simulink model "Battery_model_2D_Battery2"  (R2026a)
settings: Solver=VariableStepAuto  StopTime=10000
InitFcn:
  | %% Universal Parameters
  | 
  | Cycle_num = 1000; % number of cycles
  | 
  | Temp_state = 35;
  | 
  | 
  | SoC_state = 0.5;
  | 
  | OCV = [ 3.0025,3.4635,3.521,3.5618,3.6058,3.6426,3.6725,3.7049,3.7486,3.79951,3.8418,3.8738 ,3.9044,3.9448,3.9813,4.0222 ,4.0498,4.0658,4.0919,4.1359,4.2];
  | 
  | 
  | % Cn = 540; % As
  | Ru = 3.19; % KW^-1
  | Rc = 1.94; % KW^-1
  | Cc = 62.7; % JK^-1
  | Cs = 4.5;  % JK^-1
  | 
  | Ea = 31500;  % J * mol^-1
  | eta = 152.5; % unitless
  | Ic = 9000;   % [1/s] normalized current rate
  | Rg = 8.314;  % J / K / mol
  | z = 0.57;    % Ah power law exponent
  | 
  | 
  | 
  | %% Breakpoints
  | Temp = [5, 15, 25, 35, 45];
  | SoC  = [0, 0.05, 0.10, 0.15, 0.20, 0.25, 0.30, 0.35, 0.40, 0.45, 0.50, 0.55, 0.60, 0.65, 0.70, 0.75, 0.80, 0.85, 0.90, 0.95, 1.00];
  | 
  | %% ── CHARGING Parameters ──────────────────────────────────────────────────────
  | %% CHARGING Parameters
  | 
  | % --- R0 (charge) ---
  | R0_5_ch  = [0.10039366, 0.10039366, 0.10039366, 0.08528700, 0.07769698, 0.08283688, 0.11006698 ...
  |              0.11427069, 0.11402639, 0.11444591, 0.11423324, 0.11397462, 0.11400530, 0.11412006 ...
  |              0.11437022, 0.11469884, 0.11501972, 0.11491341, 0.11445199, 0.11423824, 0.11366247];
  | R0_15_ch  = [0.13171649, 0.13171649, 0.13171649, 0.11189655, 0.10193844, 0.10868199, 0.14440788 ...
  |              0.14992315, 0.14960263, 0.15015303, 0.14987401, 0.14953470, 0.14957496, 0.14972552 ...
  |              0.15005372, 0.15048488, 0.15090588, 0.15076639, 0.15016101, 0.14988057, 0.14912516];
  | R0_25_ch  = [0.15680534, 0.15680534, 0.15680534, 0.13321018, 0.12135528, 0.12938332, 0.17191415 ...
  |              0.17847994, 0.17809836, 0.17875361, 0.17842144, 0.17801751, 0.17806543, 0.17824467 ...
  |              0.17863539, 0.17914866, 0.17964985, 0.17948380, 0.17876310, 0.17842925, 0.17752995];
  | R0_35_ch  = [0.18293956, 0.18293956, 0.18293956, 0.15541187, 0.14158117, 0.15094720, 0.20056650 ...
  |              0.20822660, 0.20778142, 0.20854588, 0.20815835, 0.20768709, 0.20774300, 0.20795212 ...
  |              0.20840795, 0.20900677, 0.20959150, 0.20939777, 0.20855695, 0.20816746, 0.20711828];
  | R0_45_ch  = [0.20580701, 0.20580701, 0.20580701, 0.17483836, 0.15927881, 0.16981560, 0.22563732 ...
  |              0.23425492, 0.23375410, 0.23461411, 0.23417814, 0.23364798, 0.23371087, 0.23394613 ...
  |              0.23445894, 0.23513262, 0.23579043, 0.23557249, 0.23462657, 0.23418839, 0.23300807];
  | R0_ch = [R0_5_ch; R0_15_ch; R0_25_ch; R0_35_ch; R0_45_ch];
  | 
  | % --- R1 (charge) ---
  | R1_5_ch  = [0.04985788, 0.04985788, 0.05071229, 0.04160410, 0.03661133, 0.03925367, 0.05381930 ...
  |              0.05642225, 0.05603500, 0.05496214, 0.05471562, 0.05430091, 0.05382478, 0.05367572 ...
  |              0.05355262, 0.05341750, 0.05337771, 0.05361159, 0.05382278, 0.05411150, 0.05453301];
  | R1_15_ch  = [0.07380278, 0.07380278, 0.07506754, 0.06158502, 0.05419440, 0.05810577, 0.07966673 ...
  |              0.08351978, 0.08294655, 0.08135843, 0.08099351, 0.08037963, 0.07967483, 0.07945418 ...
  |              0.07927196, 0.07907196, 0.07901306, 0.07935925, 0.07967188, 0.08009926, 0.08072321];
  | R1_25_ch  = [0.09348353, 0.09348353, 0.09508555, 0.07800769, 0.06864625, 0.07360064, 0.10091119 ...
  |              0.10579172, 0.10506563, 0.10305401, 0.10259178, 0.10181420, 0.10092146, 0.10064197 ...
  |              0.10041116, 0.10015782, 0.10008321, 0.10052172, 0.10091772, 0.10145906, 0.10224939];
  | R1_35_ch  = [0.14022529, 0.14022529, 0.14262832, 0.11701153, 0.10296937, 0.11040096, 0.15136678 ...
  |              0.15868759, 0.15759844, 0.15458101, 0.15388767, 0.15272130, 0.15138219, 0.15096295 ...
  |              0.15061673, 0.15023673, 0.15012481, 0.15078258, 0.15137658, 0.15218860, 0.15337409];
  | R1_45_ch  = [0.14957364, 0.14957364, 0.15213688, 0.12481230, 0.10983399, 0.11776102, 0.16145790 ...
  |              0.16926676, 0.16810500, 0.16488641, 0.16414685, 0.16290272, 0.16147433, 0.16102715 ...
  |              0.16065785, 0.16025251, 0.16013313, 0.16083476, 0.16146835, 0.16233450, 0.16359903];
  | R1_ch = [R1_5_ch; R1_15_ch; R1_25_ch; R1_35_ch; R1_45_ch];
  | 
  | % --- C1 (charge) ---
  | C1_5_ch  = [0.09227515, 0.09227515, 0.26008928, 0.33919625, 0.34687174, 0.30913179, 0.15915764 ...
  |              0.12842562, 0.12634235, 0.13107159, 0.12652827, 0.12226041, 0.12210630, 0.12333974 ...
  |              0.12544932, 0.12714870, 0.12951385, 0.13210182, 0.12944620, 0.12631334, 0.11822176];
  | C1_15_ch  = [0.08202235, 0.08202235, 0.23119047, 0.30150778, 0.30833043, 0.27478381, 0.14147345 ...
  |              0.11415611, 0.11230431, 0.11650808, 0.11246957, 0.10867592, 0.10853893, 0.10963532 ...
  |              0.11151051, 0.11302106, 0.11512343, 0.11742384, 0.11506329, 0.11227852, 0.10508601];
  | C1_25_ch  = [0.06561788, 0.06561788, 0.18495238, 0.24120622, 0.24666435, 0.21982705, 0.11317876 ...
  |              0.09132488, 0.08984345, 0.09320646, 0.08997566, 0.08694074, 0.08683115, 0.08770826 ...
  |              0.08920840, 0.09041685, 0.09209874, 0.09393907, 0.09205063, 0.08982282, 0.08406881];
  | C1_35_ch  = [0.06151676, 0.06151676, 0.17339285, 0.22613083, 0.23124783, 0.20608786, 0.10610509 ...
  |              0.08561708, 0.08422823, 0.08738106, 0.08435218, 0.08150694, 0.08140420, 0.08222649 ...
  |              0.08363288, 0.08476580, 0.08634257, 0.08806788, 0.08629747, 0.08420889, 0.07881451];
  | C1_45_ch  = [0.04921341, 0.04921341, 0.13871428, 0.18090467, 0.18499826, 0.16487029, 0.08488407 ...
  |              0.06849366, 0.06738259, 0.06990485, 0.06748174, 0.06520555, 0.06512336, 0.06578119 ...
  |              0.06690630, 0.06781264, 0.06907406, 0.07045431, 0.06903797, 0.06736711, 0.06305160];
  | C1_ch = [C1_5_ch; C1_15_ch; C1_25_ch; C1_35_ch; C1_45_ch];
  | 
  | % --- R2 (charge) ---
  | R2_5_ch  = [0.09089386, 0.09089386, 0.09135964, 0.07050606, 0.05920502, 0.06424266, 0.09305088 ...
  |              0.09755014, 0.09580263, 0.08885962, 0.08806550, 0.08655484, 0.08420777, 0.08313697 ...
  |              0.08166340, 0.07982229, 0.07868093, 0.07801613, 0.07782377, 0.07821878, 0.07934489];
  | R2_15_ch  = [0.12119181, 0.12119181, 0.12181285, 0.09400808, 0.07894002, 0.08565687, 0.12406784 ...
  |              0.13006685, 0.12773684, 0.11847950, 0.11742067, 0.11540645, 0.11227703, 0.11084930 ...
  |              0.10888454, 0.10642972, 0.10490791, 0.10402151, 0.10376502, 0.10429170, 0.10579318];
  | R2_25_ch  = [0.12832074, 0.12832074, 0.12897831, 0.09953796, 0.08358355, 0.09069551, 0.13136595 ...
  |              0.13771784, 0.13525077, 0.12544888, 0.12432777, 0.12219507, 0.11888156, 0.11736985 ...
  |              0.11528951, 0.11269029, 0.11107897, 0.11014042, 0.10986885, 0.11042651, 0.11201631];
  | R2_35_ch  = [0.16780404, 0.16780404, 0.16866394, 0.13016503, 0.10930157, 0.11860183, 0.17178624 ...
  |              0.18009256, 0.17686640, 0.16404853, 0.16258247, 0.15979355, 0.15546051, 0.15348364 ...
  |              0.15076320, 0.14736423, 0.14525711, 0.14402978, 0.14367465, 0.14440390, 0.14648287];
  | R2_45_ch  = [0.16780404, 0.16780404, 0.16866394, 0.13016503, 0.10930157, 0.11860183, 0.17178624 ...
  |              0.18009256, 0.17686640, 0.16404853, 0.16258247, 0.15979355, 0.15546051, 0.15348364 ...
  |              0.15076320, 0.14736423, 0.14525711, 0.14402978, 0.14367465, 0.14440390, 0.14648287];
  | R2_ch = [R2_5_ch; R2_15_ch; R2_25_ch; R2_35_ch; R2_45_ch];
  | 
  | % --- C2 (charge) ---
  | C2_5_ch  = [0.00983276, 0.00983276, 0.01035565, 0.01275571, 0.01321620, 0.01188380, 0.00709573 ...
  |              0.00612936, 0.00604375, 0.00608405, 0.00594967, 0.00578324, 0.00570466, 0.00570404 ...
  |              0.00576703, 0.00583752, 0.00589611, 0.00594399, 0.00590399, 0.00585441, 0.00573186];
  | C2_15_ch  = [0.00709364, 0.00709364, 0.00747086, 0.00920233, 0.00953455, 0.00857331, 0.00511907 ...
  |              0.00442190, 0.00436013, 0.00438920, 0.00429226, 0.00417219, 0.00411551, 0.00411505 ...
  |              0.00416050, 0.00421135, 0.00425362, 0.00428816, 0.00425931, 0.00422354, 0.00413513];
  | C2_25_ch  = [0.00584182, 0.00584182, 0.00615247, 0.00757839, 0.00785198, 0.00706038, 0.00421570 ...
  |              0.00364156, 0.00359070, 0.00361464, 0.00353480, 0.00343592, 0.00338924, 0.00338887 ...
  |              0.00342629, 0.00346817, 0.00350298, 0.00353143, 0.00350767, 0.00347821, 0.00340540];
  | C2_35_ch  = [0.00496555, 0.00496555, 0.00522960, 0.00644163, 0.00667418, 0.00600132, 0.00358335 ...
  |              0.00309533, 0.00305209, 0.00307244, 0.00300458, 0.00292054, 0.00288085, 0.00288054 ...
  |              0.00291235, 0.00294795, 0.00297754, 0.00300171, 0.00298152, 0.00295648, 0.00289459];
  | C2_45_ch  = [0.00381965, 0.00381965, 0.00402277, 0.00495510, 0.00513399, 0.00461640, 0.00275642 ...
  |              0.00238102, 0.00234776, 0.00236342, 0.00231122, 0.00224657, 0.00221604, 0.00221580 ...
  |              0.00224027, 0.00226765, 0.00229041, 0.00230901, 0.00229347, 0.00227421, 0.00222661];
  | C2_ch = [C2_5_ch; C2_15_ch; C2_25_ch; C2_35_ch; C2_45_ch];
  | 
  | %% DISCHARGING Parameters
  | 
  | % --- R0 (discharge) ---
  | R0_5_dis  = [0.10974667, 0.10974667, 0.10599493, 0.10491812, 0.10459081, 0.10424192, 0.10391050 ...
  |              0.10360923, 0.10340664, 0.10367370, 0.10378809, 0.10357423, 0.10367328, 0.10392792 ...
  |              0.10349265, 0.10276346, 0.10258047, 0.10278050, 0.10278050, 0.10278050, 0.10278050];
  | R0_15_dis  = [0.15445828, 0.15445828, 0.14917805, 0.14766253, 0.14720188, 0.14671085, 0.14624440 ...
  |              0.14582040, 0.14553527, 0.14591113, 0.14607213, 0.14577114, 0.14591054, 0.14626892 ...
  |              0.14565632, 0.14463005, 0.14437252, 0.14465404, 0.14465404, 0.14465404, 0.14465404];
  | R0_25_dis  = [0.18956243, 0.18956243, 0.18308216, 0.18122220, 0.18065686, 0.18005422, 0.17948176 ...
  |              0.17896140, 0.17861147, 0.17907275, 0.17927034, 0.17890094, 0.17907203, 0.17951186 ...
  |              0.17876003, 0.17750052, 0.17718445, 0.17752995, 0.17752995, 0.17752995, 0.17752995];
  | R0_35_dis  = [0.23168742, 0.23168742, 0.22376708, 0.22149380, 0.22080283, 0.22006627, 0.21936660 ...
  |              0.21873060, 0.21830291, 0.21886669, 0.21910819, 0.21865671, 0.21886581, 0.21940339 ...
  |              0.21848448, 0.21694508, 0.21655878, 0.21698106, 0.21698106, 0.21698106, 0.21698106];
  | R0_45_dis  = [0.26064835, 0.26064835, 0.25173797, 0.24918053, 0.24840318, 0.24757455, 0.24678743 ...
  |              0.24607192, 0.24559077, 0.24622503, 0.24649672, 0.24598880, 0.24622404, 0.24682881 ...
  |              0.24579504, 0.24406321, 0.24362862, 0.24410369, 0.24410369, 0.24410369, 0.24410369];
  | R0_dis = [R0_5_dis; R0_15_dis; R0_25_dis; R0_35_dis; R0_45_dis];
  | 
  | % --- R1 (discharge) ---
  | R1_5_dis  = [0.03959912, 0.03959912, 0.03910968, 0.03839708, 0.03719962, 0.03650035, 0.03573789 ...
  |              0.03550570, 0.03600486, 0.03635088, 0.03581701, 0.03524835, 0.03530531, 0.03537131 ...
  |              0.03514362, 0.03493837, 0.03506404, 0.03578729, 0.03578729, 0.03578729, 0.03578729];
  | R1_15_dis  = [0.07199840, 0.07199840, 0.07110850, 0.06981287, 0.06763567, 0.06636428, 0.06497798 ...
  |              0.06455582, 0.06546338, 0.06609252, 0.06512184, 0.06408791, 0.06419147, 0.06431147 ...
  |              0.06389749, 0.06352431, 0.06375280, 0.06506780, 0.06506780, 0.06506780, 0.06506780];
  | R1_25_dis  = [0.11314034, 0.11314034, 0.11174193, 0.10970594, 0.10628463, 0.10428672, 0.10210826 ...
  |              0.10144487, 0.10287103, 0.10385967, 0.10233432, 0.10070958, 0.10087230, 0.10106088 ...
  |              0.10041034, 0.09982391, 0.10018297, 0.10224939, 0.10224939, 0.10224939, 0.10224939];
  | R1_35_dis  = [0.15839648, 0.15839648, 0.15643871, 0.15358832, 0.14879848, 0.14600141, 0.14295156 ...
  |              0.14202281, 0.14401945, 0.14540354, 0.14326805, 0.14099341, 0.14122123, 0.14148523 ...
  |              0.14057447, 0.13975347, 0.14025616, 0.14314915, 0.14314915, 0.14314915, 0.14314915];
  | R1_45_dis  = [0.17999600, 0.17999600, 0.17777126, 0.17453218, 0.16908919, 0.16591069, 0.16244496 ...
  |              0.16138956, 0.16365846, 0.16523129, 0.16280460, 0.16021978, 0.16047867, 0.16077867 ...
  |              0.15974372, 0.15881076, 0.15938200, 0.16266949, 0.16266949, 0.16266949, 0.16266949];
  | R1_dis = [R1_5_dis; R1_15_dis; R1_25_dis; R1_35_dis; R1_45_dis];
  | 
  | % --- C1 (discharge) ---
  | C1_5_dis  = [0.25865012, 0.25865012, 0.25495567, 0.25151206, 0.24609499, 0.23971906, 0.22786518 ...
  |              0.22182597, 0.21445199, 0.21130782, 0.20864333, 0.20649971, 0.21349917, 0.22178481 ...
  |              0.21838854, 0.21060828, 0.20687447, 0.20176513, 0.20176513, 0.20176513, 0.20176513];
  | C1_15_dis  = [0.15519007, 0.15519007, 0.15297340, 0.15090724, 0.14765700, 0.14383143, 0.13671911 ...
  |              0.13309558, 0.12867119, 0.12678469, 0.12518600, 0.12389983, 0.12809950, 0.13307089 ...
  |              0.13103312, 0.12636497, 0.12412468, 0.12105908, 0.12105908, 0.12105908, 0.12105908];
  | C1_25_dis  = [0.10777088, 0.10777088, 0.10623153, 0.10479669, 0.10253958, 0.09988294, 0.09494383 ...
  |              0.09242749, 0.08935500, 0.08804493, 0.08693472, 0.08604155, 0.08895799, 0.09241034 ...
  |              0.09099522, 0.08775345, 0.08619769, 0.08406881, 0.08406881, 0.08406881, 0.08406881];
  | C1_35_dis  = [0.07917861, 0.07917861, 0.07804765, 0.07699349, 0.07533520, 0.07338338, 0.06975465 ...
  |              0.06790591, 0.06564857, 0.06468607, 0.06387041, 0.06321420, 0.06535689, 0.06789331 ...
  |              0.06685363, 0.06447192, 0.06332892, 0.06176484, 0.06176484, 0.06176484, 0.06176484];
  | C1_45_dis  = [0.06928128, 0.06928128, 0.06829170, 0.06736930, 0.06591830, 0.06421046, 0.06103532 ...
  |              0.05941767, 0.05744250, 0.05660031, 0.05588661, 0.05531242, 0.05718728, 0.05940665 ...
  |              0.05849693, 0.05641293, 0.05541280, 0.05404423, 0.05404423, 0.05404423, 0.05404423];
  | C1_dis = [C1_5_dis; C1_15_dis; C1_25_dis; C1_35_dis; C1_45_dis];
  | 
  | % --- R2 (discharge) ---
  | R2_5_dis  = [0.08531563, 0.08531563, 0.08615528, 0.08329853, 0.07783962, 0.07496095, 0.07307666 ...
  |              0.07262795, 0.07352909, 0.07429917, 0.07148713, 0.06823238, 0.06783005, 0.06755245 ...
  |              0.06633675, 0.06454005, 0.06447191, 0.06608962, 0.06608962, 0.06608962, 0.06608962];
  | R2_15_dis  = [0.11375417, 0.11375417, 0.11487370, 0.11106470, 0.10378615, 0.09994794, 0.09743555 ...
  |              0.09683727, 0.09803879, 0.09906556, 0.09531618, 0.09097651, 0.09044007, 0.09006993 ...
  |              0.08844900, 0.08605339, 0.08596255, 0.08811950, 0.08811950, 0.08811950, 0.08811950];
  | R2_25_dis  = [0.14460276, 0.14460276, 0.14602589, 0.14118395, 0.13193155, 0.12705246, 0.12385875 ...
  |              0.12309822, 0.12462558, 0.12593079, 0.12116463, 0.11564810, 0.11496619, 0.11449568 ...
  |              0.11243517, 0.10938991, 0.10927443, 0.11201631, 0.11201631, 0.11201631, 0.11201631];
  | R2_35_dis  = [0.17063126, 0.17063126, 0.17231055, 0.16659706, 0.15567923, 0.14992191, 0.14615332 ...
  |              0.14525590, 0.14705818, 0.14859834, 0.14297426, 0.13646476, 0.13566011, 0.13510490 ...
  |              0.13267350, 0.12908009, 0.12894383, 0.13217925, 0.13217925, 0.13217925, 0.13217925];
  | R2_45_dis  = [0.17063126, 0.17063126, 0.17231055, 0.16659706, 0.15567923, 0.14992191, 0.14615332 ...
  |              0.14525590, 0.14705818, 0.14859834, 0.14297426, 0.13646476, 0.13566011, 0.13510490 ...
  |              0.13267350, 0.12908009, 0.12894383, 0.13217925, 0.13217925, 0.13217925, 0.13217925];
  | R2_dis = [R2_5_dis; R2_15_dis; R2_25_dis; R2_35_dis; R2_45_dis];
  | 
  | % --- C2 (discharge) ---
  | C2_5_dis  = [0.00775836, 0.00775836, 0.00769594, 0.00737404, 0.00681760, 0.00637471, 0.00590764 ...
  |              0.00567197, 0.00566534, 0.00568421, 0.00559762, 0.00552599, 0.00558487, 0.00564889 ...
  |              0.00560911, 0.00554423, 0.00550375, 0.00544864, 0.00544864, 0.00544864, 0.00544864];
  | C2_15_dis  = [0.00646530, 0.00646530, 0.00641328, 0.00614503, 0.00568133, 0.00531226, 0.00492304 ...
  |              0.00472664, 0.00472112, 0.00473684, 0.00466468, 0.00460499, 0.00465406, 0.00470741 ...
  |              0.00467426, 0.00462019, 0.00458646, 0.00454054, 0.00454054, 0.00454054, 0.00454054];
  | C2_25_dis  = [0.00484897, 0.00484897, 0.00480996, 0.00460877, 0.00426100, 0.00398419, 0.00369228 ...
  |              0.00354498, 0.00354084, 0.00355263, 0.00349851, 0.00345374, 0.00349054, 0.00353056 ...
  |              0.00350569, 0.00346515, 0.00343985, 0.00340540, 0.00340540, 0.00340540, 0.00340540];
  | C2_35_dis  = [0.00258612, 0.00258612, 0.00256531, 0.00245801, 0.00227253, 0.00212490, 0.00196921 ...
  |              0.00189066, 0.00188845, 0.00189474, 0.00186587, 0.00184200, 0.00186162, 0.00188296 ...
  |              0.00186970, 0.00184808, 0.00183458, 0.00181621, 0.00181621, 0.00181621, 0.00181621];
  | C2_45_dis  = [0.00149199, 0.00149199, 0.00147999, 0.00141808, 0.00131108, 0.00122591, 0.00113609 ...
  |              0.00109076, 0.00108949, 0.00109312, 0.00107646, 0.00106269, 0.00107401, 0.00108633 ...
  |              0.00107868, 0.00106620, 0.00105841, 0.00104782, 0.00104782, 0.00104782, 0.00104782];
  | C2_dis = [C2_5_dis; C2_15_dis; C2_25_dis; C2_35_dis; C2_45_dis];
model workspace (MAT data in the model file):
  C_As = 150
  Cn = 150
  I_c = 1
  I_c_full_charged = 0.0333333333333
  Tc_state = 35.0044118318
  Ts_state = 35.0027406087
  V1_state = 0.00398713164124
  V2_state = 0.00927212980774
  V_cutoff = 3
  V_max = 4.2
  current_SoC = 0.996576803874
undefined symbols (not defined in the file): V1_ini
libraries: simulink x7
(part 1 of 2)
settings Model: Creator=vatan  LastModifiedBy=beaga
settings DebuggingCC: UnderspecifiedInitializationDetection=Classic
settings SimscapeCC: SimscapeNominalValues="[{\"value\":\"1\",\"unit\":\"A\"},{\"value\":\"1\",\"unit\":\"bar\"},{\"value\":\"1\",\"unit\":\"cm^2\"},{\"value\":\"1\",\"unit\":\"cm^3/s\"},{\"value\":\"1\",\"unit\":\"kJ/kg\"},{\"value\":\"1\",\"unit\":\"kW\"},{\"value\":\"1\",\"unit\":\"l\"},{\"value\":\"1\",\"unit\":\"N\"},{\"value\":\"1\",\"unit\":\"N*m\"},{\"value\":\"1\",\"unit\":\"V\"}]"  SimscapeLogType=none  SimscapeLogDataHistory=5000.0

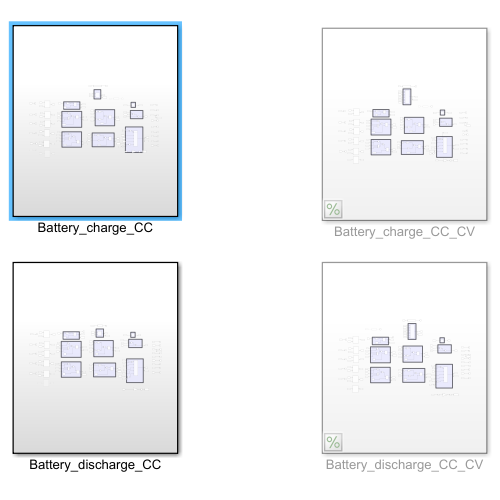
[thumbnail: Simulink's stored preview of the top-level diagram]
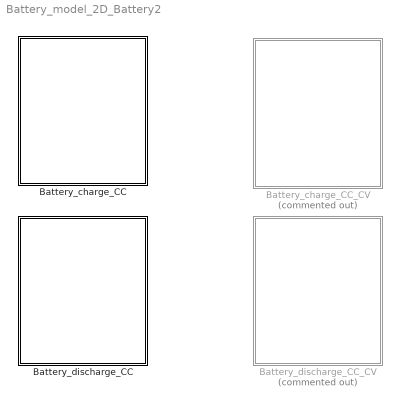
== system Battery_model_2D_Battery2 ==
  Battery_charge_CC : Subsystem
  Battery_charge_CC_CV : Subsystem  Commented=on
  Battery_discharge_CC : Subsystem
  Battery_discharge_CC_CV : Subsystem  Commented=on

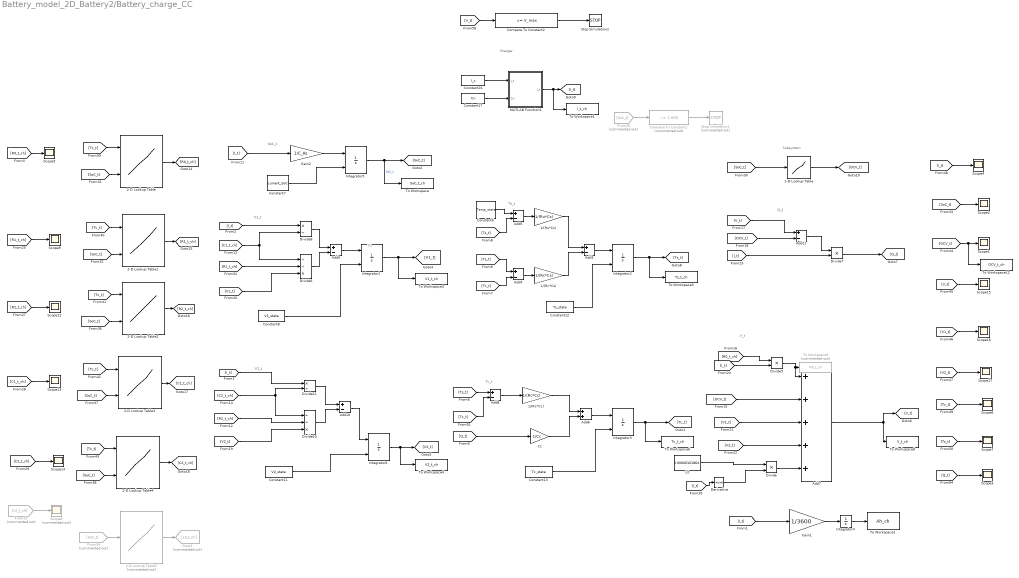
== system Battery_model_2D_Battery2/Battery_charge_CC ==
  note: Subsystem
  note: Tc_t
  note: Ts_t
  note: V_t
  note: V2_t
  note: V1_t
  note: SoC_t
  note: V1
  note: Q_t
  note: Charger
  1-D Lookup Table : Lookup_n-D  NumberOfTableDimensions=1  BreakpointsForDimension1=SoC  BreakpointsForDimension2=Temp  Table=OCV  InternalRulePriority=Speed  RndMeth=Simplest
  1/(Rc*Cc) : Gain  Gain=1/(Rc*Cc)
  1/(Rc*Cs) : Gain  Gain=1/(Rc*Cs)
  1/(Ru*Cs) : Gain  Gain=1/(Ru*Cs)
  2-D Lookup Table : Lookup_n-D  BreakpointsForDimension1=Temp  BreakpointsForDimension2=SoC  Table=R0_ch  InternalRulePriority=Speed  RndMeth=Simplest
      settings: InputPortMap=u0,u1
  2-D Lookup Table1 : Lookup_n-D  BreakpointsForDimension1=Temp  BreakpointsForDimension2=SoC  Table=R1_ch  InternalRulePriority=Speed  RndMeth=Simplest
      settings: InputPortMap=u0,u1
  2-D Lookup Table2 : Lookup_n-D  BreakpointsForDimension1=Temp  BreakpointsForDimension2=SoC  Table=R2_ch  InternalRulePriority=Speed  RndMeth=Simplest
      settings: InputPortMap=u0,u1
  2-D Lookup Table3 : Lookup_n-D  BreakpointsForDimension1=Temp  BreakpointsForDimension2=SoC  Table=C1_ch  InternalRulePriority=Speed  RndMeth=Simplest
      settings: InputPortMap=u0,u1
  2-D Lookup Table4 : Lookup_n-D  BreakpointsForDimension1=Temp  BreakpointsForDimension2=SoC  Table=C2_ch  InternalRulePriority=Speed  RndMeth=Simplest
      settings: InputPortMap=u0,u1
  2-D Lookup Table5 : Lookup_n-D  Commented=on  NumberOfTableDimensions=1  BreakpointsForDimension1=Temp  BreakpointsForDimension2=SoC  Table=C2_ch  InternalRulePriority=Speed  RndMeth=Simplest
  Add{3..5,8..11} (7 alike) : Sum  Inputs=+-
  Add6 : Sum
  Add7 : Sum  Inputs=+++++
  Cc : Gain  Gain=1/Cc
  Compare To Constant1 : simulink/Logic and Bit Operations/Compare To Constant  Commented=on  relop=~=  const=1.000  OutDataTypeStr=boolean
  Compare To Constant2 : simulink/Logic and Bit Operations/Compare To Constant  relop=>=  const=V_max  OutDataTypeStr=boolean
  Constant11 : Constant  Value=V2_state
  Constant12 : Constant  Value=Ts_state
  Constant13 : Constant  Value=Tc_state
  Constant16 : Constant  Value=I_c
  Constant17 : Constant  Value=Cn
  Constant6 : Constant  Value=Temp_state
  Constant7 : Constant  Value=current_SoC
  Constant8 : Constant  Value=V1_state
  Derivative : Derivative
  Divide : Product  Inputs=**
  Divide10 : Product  Inputs=//*
  Divide11 : Product  Inputs=*/
  Divide5 : Product  Inputs=**
  Divide6 : Product  Inputs=//*
  Divide7 : Product  Inputs=**
  Divide8 : Product  Inputs=*/
  From26 : From  Commented=on  GotoTag=SoC_t
  From34 : From  Commented=on  GotoTag=SoC_t
  From53 : From  Commented=on  GotoTag=L0_t_ch
  Gain1 : Gain  Gain=1/3600
  Gain2 : Gain  Gain=1/C_As
  Goto3 : Goto  Commented=on  GotoTag=L0_t_ch
  Integrator{1..3,6} (4 alike) : Integrator  InitialConditionSource=external
  Integrator4 : Integrator
  Integrator5 : Integrator  InitialConditionSource=external  InitialCondition=V1_ini
  L0 : Constant  Value=0.00000101864
  MATLAB Function4 : MATLAB Function  TreatAsAtomicUnit=on
  Scope{1..7,9,12..17} (14 alike) : Scope
      Scope1 settings: ActiveDisplayYMinimum=2.2604  ActiveDisplayYMaximum=3.6664  DataLoggingVariableName=ScopeData7
      Scope12 settings: ActiveDisplayYMinimum=0.00751  ActiveDisplayYMaximum=0.04204  DataLoggingVariableName=ScopeData3
      Scope13 settings: ActiveDisplayYMinimum=1446.0874  ActiveDisplayYMaximum=2982.5444  DataLoggingVariableName=ScopeData4
      Scope14 settings: ActiveDisplayYMinimum=14445.3812  ActiveDisplayYMaximum=112360.8817  DataLoggingVariableName=ScopeData5
      Scope15 settings: ActiveDisplayYMinimum=2.15  ActiveDisplayYMaximum=4.15  DataLoggingVariableName=ScopeData8
      Scope16 settings: ActiveDisplayYMinimum=-0.00306  ActiveDisplayYMaximum=0.0275  DataLoggingVariableName=ScopeData9
      Scope17 settings: ActiveDisplayYMinimum=-0.00274  ActiveDisplayYMaximum=0.02463  DataLoggingVariableName=ScopeData10
      Scope2 settings: ActiveDisplayYMinimum=0.0058466  ActiveDisplayYMaximum=0.025847  DataLoggingVariableName=ScopeData6
      Scope3 settings: ActiveDisplayYMinimum=-7.8351  ActiveDisplayYMaximum=6.6118  DataLoggingVariableName=ScopeData14
      Scope4 settings: ActiveDisplayYMinimum=0.049838  ActiveDisplayYMaximum=0.24984  DataLoggingVariableName=ScopeData11
      Scope5 settings: ActiveDisplayYMinimum=0.00753  ActiveDisplayYMaximum=0.01894
      Scope6 settings: ActiveDisplayYMinimum=24.9953  ActiveDisplayYMaximum=44.9953  DataLoggingVariableName=ScopeData12
      Scope7 settings: ActiveDisplayYMinimum=-5.0616  ActiveDisplayYMaximum=45.5546  DataLoggingVariableName=ScopeData13
      Scope9 settings: ActiveDisplayYMinimum=0.00821  ActiveDisplayYMaximum=0.03092  DataLoggingVariableName=ScopeData2
  Scope8 : Scope  Commented=on
      settings: ActiveDisplayYMinimum=14445.3812  ActiveDisplayYMaximum=112360.8817  DataLoggingVariableName=ScopeData24
  Stop Simulation1 : Stop  Commented=on
  Stop Simulation2 : Stop
  To Workspace : ToWorkspace  VariableName=SoC_t_ch  SampleTime=-1
      settings: Save2DSignal=2-D array (concatenate along first dimension)
  To Workspace1 : ToWorkspace  VariableName=I_t_ch  SaveFormat=Timeseries  SampleTime=-1
      settings: Save2DSignal=2-D array (concatenate along first dimension)
  To Workspace12 : ToWorkspace  VariableName=OCV_t_ch  SampleTime=-1
      settings: Save2DSignal=2-D array (concatenate along first dimension)
  To Workspace2 : ToWorkspace  VariableName=Ah_ch  SampleTime=-1
      settings: Save2DSignal=2-D array (concatenate along first dimension)
  To Workspace3 : ToWorkspace  VariableName=V1_t_ch  SampleTime=-1
      settings: Save2DSignal=2-D array (concatenate along first dimension)
  To Workspace4 : ToWorkspace  VariableName=V2_t_ch  SampleTime=-1
      settings: Save2DSignal=2-D array (concatenate along first dimension)
  To Workspace5 : ToWorkspace  VariableName=Ts_t_ch  SampleTime=-1
      settings: Save2DSignal=2-D array (concatenate along first dimension)
  To Workspace6 : ToWorkspace  VariableName=Tc_t_ch  SampleTime=-1
      settings: Save2DSignal=2-D array (concatenate along first dimension)
  To Workspace8 : ToWorkspace  VariableName=V_t_ch  SaveFormat=Timeseries  SampleTime=-1
      settings: Save2DSignal=2-D array (concatenate along first dimension)
  To Workspace9 : ToWorkspace  Commented=on  VariableName=R0_I_ch  SampleTime=-1
      settings: Save2DSignal=2-D array (concatenate along first dimension)
  wires:
  Divide10/1 -> Add10/2
  Add5/1 -> 1/(Ru*Cs)/1
  Add11/1 -> Divide7/1
  [Tc_t] -> Add4/2
  1/(Rc*Cc)/1 -> Add6/1
  [V2_t] -> Add7/4
  Divide5/1 -> Add7/1, To Workspace9/1
  Add4/1 -> 1/(Rc*Cs)/1
  Divide6/1 -> Add9/2
  [I_t] -> Divide11/1
  [Tc_t] -> 2-D Lookup Table2/1
  Cc/1 -> Add6/2
  [Tc_t] -> 2-D Lookup Table/1
  Divide7/1 -> [Q_t]
  1-D Lookup Table/1 -> [OCV_t]
  [SoC_t] -> 2-D Lookup Table1/2
  2-D Lookup Table3/1 -> [C1_t_ch]
  [V2_t] -> Scope17/1
  Add9/1 -> Integrator1/1
  2-D Lookup Table/1 -> [R0_t_ch]
  [Ts_t] -> Scope7/1
  [I_t] -> Scope4/1
  [V2_t] -> Divide10/3
  [R1_t_ch] -> Scope9/1
  Add10/1 -> Integrator6/1
  2-D Lookup Table4/1 -> [C2_t_ch]
  [SoC_t] -> 1-D Lookup Table/1
  [R0_t_ch] -> Scope5/1
  [SoC_t] -> 2-D Lookup Table/2
  [R0_t_ch] -> Divide5/1
  [I_t] -> Divide7/2
  [V1_t] -> Scope16/1
  [C2_t_ch] -> Divide10/1, Divide11/2
  Add3/1 -> Integrator2/1
  [V_t] -> Add11/1
  [Q_t] -> Scope3/1
  [I_t] -> Divide5/2
  [SoC_t] -> 2-D Lookup Table3/2
  1/(Rc*Cs)/1 -> Add3/2
  [OCV_t] -> To Workspace12/1, Scope1/1
  [C1_t_ch] -> Scope13/1
  [Tc_t] -> Scope6/1
  Divide8/1 -> Add9/1
  [OCV_t] -> Add11/2
  [V1_t] -> Divide6/3
  [Ts_t] -> Add4/1
  [Tc_t] -> 2-D Lookup Table1/1
  [C1_t_ch] -> Divide8/2, Divide6/1
  [Tc_t] -> 2-D Lookup Table3/1
  Gain2/1 -> Integrator5/1
  Add8/1 -> 1/(Rc*Cc)/1
  [R1_t_ch] -> Divide6/2
  [R2_t_ch] -> Scope12/1
  [Q_t] -> Cc/1
  Add6/1 -> Integrator3/1
  [R2_t_ch] -> Divide10/2
  [Ts_t] -> Add8/1
  2-D Lookup Table2/1 -> [R2_t_ch]
  Divide11/1 -> Add10/1
  [C2_t_ch] -> Scope14/1
  Add7/1 -> To Workspace8/1, [V_t]
  [SoC_t] -> 2-D Lookup Table2/2
  Integrator3/1 -> To Workspace6/1, [Tc_t]
  [Ts_t] -> Add5/2
  [Tc_t] -> Add8/2
  [I_t] -> Divide8/1
  Integrator6/1 -> To Workspace4/1, [V2_t]
  Integrator5/1 -> To Workspace/1, [SoC_t]  "SoC_t"
  Integrator1/1 -> To Workspace3/1, [V1_t]
  [SoC_t] -> Scope2/1
  Constant6/1 -> Add5/1
  2-D Lookup Table1/1 -> [R1_t_ch]
  [V_t] -> Scope15/1
  [SoC_t] -> 2-D Lookup Table4/2
  1/(Ru*Cs)/1 -> Add3/1
  [I_t] -> Gain2/1
  [Tc_t] -> 2-D Lookup Table4/1
  [OCV_t] -> Add7/2
  [V1_t] -> Add7/3
  [I_t] -> Gain1/1
  Integrator4/1 -> To Workspace2/1
  Gain1/1 -> Integrator4/1
  Integrator2/1 -> To Workspace5/1, [Ts_t]
  From26/1 -> Compare To Constant1/1
  Compare To Constant1/1 -> Stop Simulation1/1
  Constant12/1 -> Integrator2/2
  Constant8/1 -> Integrator1/2
  Constant11/1 -> Integrator6/2
  Constant13/1 -> Integrator3/2
  Constant16/1 -> MATLAB Function4/1(I_c)
  Constant17/1 -> MATLAB Function4/2(Cn)
  [V_t] -> Compare To Constant2/1
  Compare To Constant2/1 -> Stop Simulation2/1
  MATLAB Function4/1(I_t) -> To Workspace1/1, [I_t]
  Constant7/1 -> Integrator5/2
  From34/1 -> 2-D Lookup Table5/1
  2-D Lookup Table5/1 -> Goto3/1
  From53/1 -> Scope8/1
  [I_t] -> Derivative/1
  L0/1 -> Divide/1
  Derivative/1 -> Divide/2
  Divide/1 -> Add7/5

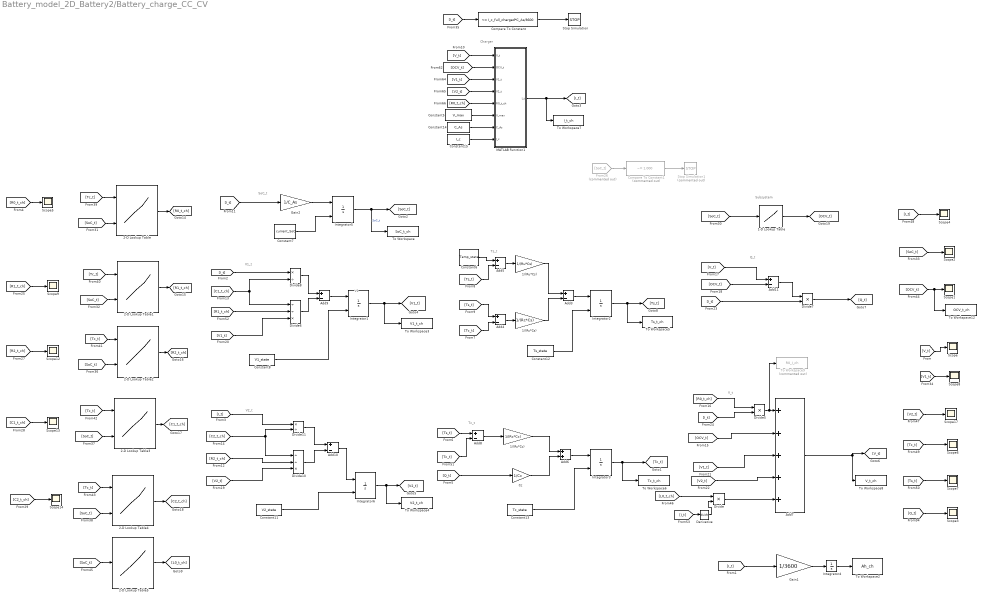
== system Battery_model_2D_Battery2/Battery_charge_CC_CV ==
  note: Subsystem
  note: Tc_t
  note: Ts_t
  note: V_t
  note: V2_t
  note: V1_t
  note: SoC_t
  note: V1
  note: Q_t
  note: Charger
  1-D Lookup Table : Lookup_n-D  NumberOfTableDimensions=1  BreakpointsForDimension1=SoC  BreakpointsForDimension2=Temp  Table=OCV  InternalRulePriority=Speed  RndMeth=Simplest
  1/(Rc*Cc) : Gain  Gain=1/(Rc*Cc)
  1/(Rc*Cs) : Gain  Gain=1/(Rc*Cs)
  1/(Ru*Cs) : Gain  Gain=1/(Ru*Cs)
  2-D Lookup Table : Lookup_n-D  BreakpointsForDimension1=Temp  BreakpointsForDimension2=SoC  Table=R0_ch  InternalRulePriority=Speed  RndMeth=Simplest
      settings: InputPortMap=u0,u1
  2-D Lookup Table1 : Lookup_n-D  BreakpointsForDimension1=Temp  BreakpointsForDimension2=SoC  Table=R1_ch  InternalRulePriority=Speed  RndMeth=Simplest
      settings: InputPortMap=u0,u1
  2-D Lookup Table2 : Lookup_n-D  BreakpointsForDimension1=Temp  BreakpointsForDimension2=SoC  Table=R2_ch  InternalRulePriority=Speed  RndMeth=Simplest
      settings: InputPortMap=u0,u1
  2-D Lookup Table3 : Lookup_n-D  BreakpointsForDimension1=Temp  BreakpointsForDimension2=SoC  Table=C1_ch  InternalRulePriority=Speed  RndMeth=Simplest
      settings: InputPortMap=u0,u1
  2-D Lookup Table4 : Lookup_n-D  BreakpointsForDimension1=Temp  BreakpointsForDimension2=SoC  Table=C2_ch  InternalRulePriority=Speed  RndMeth=Simplest
      settings: InputPortMap=u0,u1
  2-D Lookup Table5 : Lookup_n-D  NumberOfTableDimensions=1  BreakpointsForDimension1=Temp  BreakpointsForDimension2=SoC  Table=C2_ch  InternalRulePriority=Speed  RndMeth=Simplest
  Add{3..5,8..11} (7 alike) : Sum  Inputs=+-
  Add6 : Sum
  Add7 : Sum  Inputs=+++++
  Cc : Gain  Gain=1/Cc
  Compare To Constant : simulink/Logic and Bit Operations/Compare To Constant  relop=<=  const=I_c_full_charged*C_As/3600  OutDataTypeStr=boolean
  Compare To Constant1 : simulink/Logic and Bit Operations/Compare To Constant  Commented=on  relop=~=  const=1.000  OutDataTypeStr=boolean
  Constant11 : Constant  Value=V2_state
  Constant12 : Constant  Value=Ts_state
  Constant13 : Constant  Value=Tc_state
  Constant14 : Constant  Value=C_As
  Constant15 : Constant  Value=I_c
  Constant5 : Constant  Value=V_max
  Constant6 : Constant  Value=Temp_state
  Constant7 : Constant  Value=current_SoC
  Constant8 : Constant  Value=V1_state
  Derivative : Derivative
  Divide : Product  Inputs=**
  Divide10 : Product  Inputs=//*
  Divide11 : Product  Inputs=*/
  Divide5 : Product  Inputs=**
  Divide6 : Product  Inputs=//*
  Divide7 : Product  Inputs=**
  Divide8 : Product  Inputs=*/
  From26 : From  Commented=on  GotoTag=SoC_t
  Gain1 : Gain  Gain=1/3600
  Gain2 : Gain  Gain=1/C_As
  Integrator{1..3,6} (4 alike) : Integrator  InitialConditionSource=external
  Integrator4 : Integrator
  Integrator5 : Integrator  InitialConditionSource=external  InitialCondition=V1_ini
  MATLAB Function1 : MATLAB Function  TreatAsAtomicUnit=on
  Scope{,1..9,12..14,17} (14 alike) : Scope
      Scope settings: ActiveDisplayYMinimum=2.85883  ActiveDisplayYMaximum=4.3268
      Scope1 settings: ActiveDisplayYMinimum=2.85734  ActiveDisplayYMaximum=4.32322  DataLoggingVariableName=ScopeData7
      Scope12 settings: ActiveDisplayYMinimum=0.00751  ActiveDisplayYMaximum=0.04204  DataLoggingVariableName=ScopeData3
      Scope13 settings: ActiveDisplayYMinimum=1446.0874  ActiveDisplayYMaximum=2982.5444  DataLoggingVariableName=ScopeData4
      Scope14 settings: ActiveDisplayYMinimum=14445.3812  ActiveDisplayYMaximum=112360.8817  DataLoggingVariableName=ScopeData5
      Scope17 settings: ActiveDisplayYMinimum=-0.00038  ActiveDisplayYMaximum=0.00342  DataLoggingVariableName=ScopeData10
      Scope2 settings: ActiveDisplayYMinimum=0.00585  ActiveDisplayYMaximum=0.02585  DataLoggingVariableName=ScopeData6
      Scope3 settings: ActiveDisplayYMinimum=-0.00017  ActiveDisplayYMaximum=0.0017  DataLoggingVariableName=ScopeData14
      Scope4 settings: ActiveDisplayYMinimum=0.049838  ActiveDisplayYMaximum=0.24984  DataLoggingVariableName=ScopeData11
      Scope5 settings: ActiveDisplayYMinimum=0.00753  ActiveDisplayYMaximum=0.01894
      Scope6 settings: ActiveDisplayYMinimum=23.74914  ActiveDisplayYMaximum=36.2577  DataLoggingVariableName=ScopeData12
      Scope7 settings: ActiveDisplayYMinimum=23.74954  ActiveDisplayYMaximum=36.2541  DataLoggingVariableName=ScopeData13
      Scope8 settings: DataLoggingVariableName=ScopeData2
      Scope9 settings: ActiveDisplayYMinimum=0.00821  ActiveDisplayYMaximum=0.03092  DataLoggingVariableName=ScopeData2
  Stop Simulation : Stop
  Stop Simulation1 : Stop  Commented=on
  To Workspace : ToWorkspace  VariableName=SoC_t_ch  SampleTime=-1
      settings: Save2DSignal=2-D array (concatenate along first dimension)
  To Workspace12 : ToWorkspace  VariableName=OCV_t_ch  SampleTime=-1
      settings: Save2DSignal=2-D array (concatenate along first dimension)
  To Workspace2 : ToWorkspace  VariableName=Ah_ch  SampleTime=-1
      settings: Save2DSignal=2-D array (concatenate along first dimension)
  To Workspace3 : ToWorkspace  VariableName=V1_t_ch  SampleTime=-1
      settings: Save2DSignal=2-D array (concatenate along first dimension)
  To Workspace4 : ToWorkspace  VariableName=V2_t_ch  SampleTime=-1
      settings: Save2DSignal=2-D array (concatenate along first dimension)
  To Workspace5 : ToWorkspace  VariableName=Ts_t_ch  SampleTime=-1
      settings: Save2DSignal=2-D array (concatenate along first dimension)
  To Workspace6 : ToWorkspace  VariableName=Tc_t_ch  SampleTime=-1
      settings: Save2DSignal=2-D array (concatenate along first dimension)
  To Workspace7 : ToWorkspace  VariableName=I_t_ch  SaveFormat=Timeseries  SampleTime=-1
  To Workspace8 : ToWorkspace  VariableName=V_t_ch  SaveFormat=Timeseries  SampleTime=-1
      settings: Save2DSignal=2-D array (concatenate along first dimension)
  To Workspace9 : ToWorkspace  Commented=on  VariableName=R0_I_ch  SampleTime=-1
      settings: Save2DSignal=2-D array (concatenate along first dimension)
  wires:
  Divide10/1 -> Add10/2
  Add5/1 -> 1/(Ru*Cs)/1
  Add11/1 -> Divide7/1
  [Tc_t] -> Add4/2
  1/(Rc*Cc)/1 -> Add6/1
  [V2_t] -> Add7/4
  Divide5/1 -> To Workspace9/1, Add7/1
  Add4/1 -> 1/(Rc*Cs)/1
  Divide6/1 -> Add9/2
  [I_t] -> Divide11/1
  [Tc_t] -> 2-D Lookup Table2/1
  Cc/1 -> Add6/2
  [Tc_t] -> 2-D Lookup Table/1
  Divide7/1 -> [Q_t]
  1-D Lookup Table/1 -> [OCV_t]
  [SoC_t] -> 2-D Lookup Table1/2
  2-D Lookup Table3/1 -> [C1_t_ch]
  [V2_t] -> Scope17/1
  Add9/1 -> Integrator1/1
  2-D Lookup Table/1 -> [R0_t_ch]
  [Ts_t] -> Scope7/1
  [I_t] -> Scope4/1
  [V2_t] -> Divide10/3
  [R1_t_ch] -> Scope9/1
  Add10/1 -> Integrator6/1
  2-D Lookup Table4/1 -> [C2_t_ch]
  [SoC_t] -> 1-D Lookup Table/1
  [R0_t_ch] -> Scope5/1
  [SoC_t] -> 2-D Lookup Table/2
  [R0_t_ch] -> Divide5/1
  [I_t] -> Divide7/2
  [C2_t_ch] -> Divide10/1, Divide11/2
  Add3/1 -> Integrator2/1
  [V_t] -> Add11/1
  [Q_t] -> Scope3/1
  [I_t] -> Divide5/2
  [SoC_t] -> 2-D Lookup Table3/2
  1/(Rc*Cs)/1 -> Add3/2
  [OCV_t] -> To Workspace12/1, Scope1/1
  [C1_t_ch] -> Scope13/1
  [Tc_t] -> Scope6/1
  Divide8/1 -> Add9/1
  [OCV_t] -> Add11/2
  [V1_t] -> Divide6/3
  [Ts_t] -> Add4/1
  [Tc_t] -> 2-D Lookup Table1/1
  [C1_t_ch] -> Divide8/2, Divide6/1
  [Tc_t] -> 2-D Lookup Table3/1
  Gain2/1 -> Integrator5/1
  Add8/1 -> 1/(Rc*Cc)/1
  [R1_t_ch] -> Divide6/2
  [R2_t_ch] -> Scope12/1
  [Q_t] -> Cc/1
  Add6/1 -> Integrator3/1
  [R2_t_ch] -> Divide10/2
  [Ts_t] -> Add8/1
  2-D Lookup Table2/1 -> [R2_t_ch]
  Divide11/1 -> Add10/1
  [C2_t_ch] -> Scope14/1
  Add7/1 -> [V_t], To Workspace8/1
  [SoC_t] -> 2-D Lookup Table2/2
  Integrator3/1 -> To Workspace6/1, [Tc_t]
  [Ts_t] -> Add5/2
  [Tc_t] -> Add8/2
  [I_t] -> Divide8/1
  Integrator6/1 -> To Workspace4/1, [V2_t]
  Integrator5/1 -> To Workspace/1, [SoC_t]  "SoC_t"
  Integrator1/1 -> To Workspace3/1, [V1_t]
  [SoC_t] -> Scope2/1
  Constant6/1 -> Add5/1
  2-D Lookup Table1/1 -> [R1_t_ch]
  [SoC_t] -> 2-D Lookup Table4/2
  1/(Ru*Cs)/1 -> Add3/1
  [I_t] -> Gain2/1
  [Tc_t] -> 2-D Lookup Table4/1
  [OCV_t] -> Add7/2
  [V1_t] -> Add7/3
  [I_t] -> Gain1/1
  Integrator4/1 -> To Workspace2/1
  Gain1/1 -> Integrator4/1
  Integrator2/1 -> To Workspace5/1, [Ts_t]
  [I_t] -> Compare To Constant/1
  Compare To Constant/1 -> Stop Simulation/1
  [V1_t] -> MATLAB Function1/3(V1_t)
  [R0_t_ch] -> MATLAB Function1/5(R0_t_ch)
  [OCV_t] -> MATLAB Function1/2(OCV_t)
  [V_t] -> MATLAB Function1/1(V_t)
  [V2_t] -> MATLAB Function1/4(V2_t)
  From26/1 -> Compare To Constant1/1
  Compare To Constant1/1 -> Stop Simulation1/1
  Constant12/1 -> Integrator2/2
  Constant8/1 -> Integrator1/2
  Constant11/1 -> Integrator6/2
  Constant13/1 -> Integrator3/2
  Constant14/1 -> MATLAB Function1/7(C_As)
  Constant15/1 -> MATLAB Function1/8(I_c)
  Constant5/1 -> MATLAB Function1/6(V_max)
  MATLAB Function1/1(I_t) -> To Workspace7/1, [I_t]
  Constant7/1 -> Integrator5/2
  [V_t] -> Scope/1
  [V1_t] -> Scope8/1
  [SoC_t] -> 2-D Lookup Table5/1
  2-D Lookup Table5/1 -> [L0_t_ch]
  Derivative/1 -> Divide/2
  [L0_t_ch] -> Divide/1
  [I_t] -> Derivative/1
  Divide/1 -> Add7/5

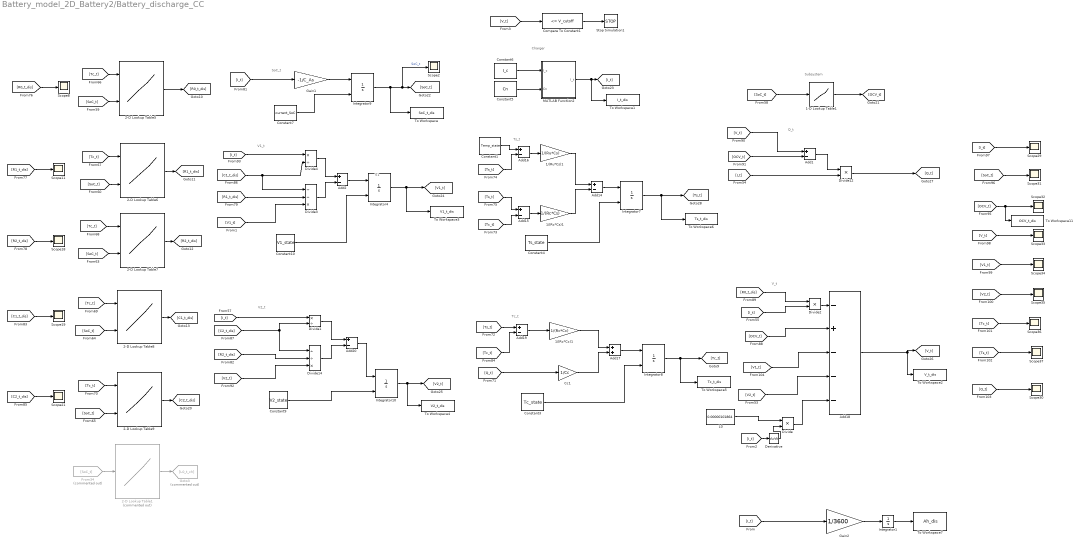
== system Battery_model_2D_Battery2/Battery_discharge_CC ==
  note: Q_t
  note: V1
  note: SoC_t
  note: V1_t
  note: V2_t
  note: V_t
  note: Ts_t
  note: Tc_t
  note: Subsystem
  note: Charger
  1-D Lookup Table1 : Lookup_n-D  NumberOfTableDimensions=1  BreakpointsForDimension1=SoC  BreakpointsForDimension2=Temp  Table=OCV  InternalRulePriority=Speed  RndMeth=Simplest
  1/(Rc*Cc)1 : Gain  Gain=1/(Rc*Cc)
  1/(Rc*Cs)1 : Gain  Gain=1/(Rc*Cs)
  1/(Ru*Cs)1 : Gain  Gain=1/(Ru*Cs)
  2-D Lookup Table1 : Lookup_n-D  Commented=on  NumberOfTableDimensions=1  BreakpointsForDimension1=Temp  BreakpointsForDimension2=SoC  Table=C2_ch  InternalRulePriority=Speed  RndMeth=Simplest
  2-D Lookup Table5 : Lookup_n-D  BreakpointsForDimension1=Temp  BreakpointsForDimension2=SoC  Table=R0_dis  InternalRulePriority=Speed  RndMeth=Simplest
      settings: InputPortMap=u0,u1
  2-D Lookup Table6 : Lookup_n-D  BreakpointsForDimension1=Temp  BreakpointsForDimension2=SoC  Table=R1_dis  InternalRulePriority=Speed  RndMeth=Simplest
      settings: InputPortMap=u0,u1
  2-D Lookup Table7 : Lookup_n-D  BreakpointsForDimension1=Temp  BreakpointsForDimension2=SoC  Table=R2_dis  InternalRulePriority=Speed  RndMeth=Simplest
      settings: InputPortMap=u0,u1
  2-D Lookup Table8 : Lookup_n-D  BreakpointsForDimension1=Temp  BreakpointsForDimension2=SoC  Table=C1_dis  InternalRulePriority=Speed  RndMeth=Simplest
      settings: InputPortMap=u0,u1
  2-D Lookup Table9 : Lookup_n-D  BreakpointsForDimension1=Temp  BreakpointsForDimension2=SoC  Table=C2_dis  InternalRulePriority=Speed  RndMeth=Simplest
      settings: InputPortMap=u0,u1
  Add{1..2,14..16,19..20} (7 alike) : Sum  Inputs=+-
  Add17 : Sum
  Add18 : Sum  Inputs=-+---
  Cc1 : Gain  Gain=1/Cc
  Compare To Constant1 : simulink/Logic and Bit Operations/Compare To Constant  relop=<=  const=V_cutoff  OutDataTypeStr=boolean
  Constant1 : Constant  Value=Temp_state
  Constant10 : Constant  Value=V1_state
  Constant3 : Constant  Value=Tc_state
  Constant4 : Constant  Value=Ts_state
  Constant5 : Constant  Value=Cn
  Constant6 : Constant  Value=I_c
  Constant7 : Constant  Value=current_SoC
  Constant9 : Constant  Value=V2_state
  Derivative : Derivative
  Divide : Product  Inputs=**
  Divide1 : Product  Inputs=*/
  Divide12 : Product  Inputs=**
  Divide14 : Product  Inputs=//*
  Divide2 : Product  Inputs=**
  Divide3 : Product  Inputs=//*
  Divide4 : Product  Inputs=*/
  From34 : From  Commented=on  GotoTag=SoC_t
  Gain1 : Gain  Gain=-1/C_As
  Gain2 : Gain  Gain=1/3600
  Goto3 : Goto  Commented=on  GotoTag=L0_t_ch
  Integrator1 : Integrator
  Integrator{4,7..8,10} (4 alike) : Integrator  InitialConditionSource=external
  Integrator9 : Integrator  InitialConditionSource=external  InitialCondition=V1_ini
  L0 : Constant  Value=0.00000101864
  MATLAB Function2 : MATLAB Function  TreatAsAtomicUnit=on
  Scope{2,8,11,18..19,21,29..37} (15 alike) : Scope
      Scope11 settings: ActiveDisplayYMinimum=-0.125  ActiveDisplayYMaximum=1.125  DataLoggingVariableName=ScopeData7
      Scope18 settings: ActiveDisplayYMinimum=-0.125  ActiveDisplayYMaximum=1.125  DataLoggingVariableName=ScopeData8
      Scope19 settings: ActiveDisplayYMinimum=-0.125  ActiveDisplayYMaximum=1.125  DataLoggingVariableName=ScopeData9
      Scope2 settings: ActiveDisplayYMinimum=-1  ActiveDisplayYMaximum=1
      Scope21 settings: ActiveDisplayYMinimum=-0.125  ActiveDisplayYMaximum=1.125  DataLoggingVariableName=ScopeData10
      Scope29 settings: ActiveDisplayYMinimum=-0.012532  ActiveDisplayYMaximum=0.16806  DataLoggingVariableName=ScopeData15
      Scope30 settings: ActiveDisplayYMinimum=-0.17004  ActiveDisplayYMaximum=1.5304  DataLoggingVariableName=ScopeData23
      Scope31 settings: ActiveDisplayYMinimum=-0.037306  ActiveDisplayYMaximum=0.031954  DataLoggingVariableName=ScopeData16
      Scope32 settings: ActiveDisplayYMinimum=2.8624  ActiveDisplayYMaximum=4.3229  DataLoggingVariableName=ScopeData17
      Scope33 settings: ActiveDisplayYMinimum=2.8623  ActiveDisplayYMaximum=3.1057  DataLoggingVariableName=ScopeData18
      Scope34 settings: ActiveDisplayYMinimum=4.0625E-5  ActiveDisplayYMaximum=0.012439  DataLoggingVariableName=ScopeData19
      Scope35 settings: ActiveDisplayYMinimum=0.00072388  ActiveDisplayYMaximum=0.0085292  DataLoggingVariableName=ScopeData20
      Scope36 settings: ActiveDisplayYMinimum=-4.1824  ActiveDisplayYMaximum=42.6414  DataLoggingVariableName=ScopeData21
      Scope37 settings: ActiveDisplayYMinimum=2.2586  ActiveDisplayYMaximum=3.6824  DataLoggingVariableName=ScopeData22
      Scope8 settings: ActiveDisplayYMinimum=-0.125  ActiveDisplayYMaximum=1.125  DataLoggingVariableName=ScopeData6
  Stop Simulation1 : Stop
  To Workspace : ToWorkspace  VariableName=SoC_t_dis  SampleTime=-1
      settings: Save2DSignal=2-D array (concatenate along first dimension)
  To Workspace1 : ToWorkspace  VariableName=I_t_dis  SaveFormat=Timeseries  SampleTime=-1
  To Workspace11 : ToWorkspace  VariableName=OCV_t_dis  SaveFormat=Timeseries  SampleTime=-1
  To Workspace2 : ToWorkspace  VariableName=V_t_dis  SaveFormat=Timeseries  SampleTime=-1
  To Workspace3 : ToWorkspace  VariableName=V1_t_dis  SampleTime=-1
      settings: Save2DSignal=2-D array (concatenate along first dimension)
  To Workspace4 : ToWorkspace  VariableName=V2_t_dis  SampleTime=-1
      settings: Save2DSignal=2-D array (concatenate along first dimension)
  To Workspace5 : ToWorkspace  VariableName=Tc_t_dis  SampleTime=-1
      settings: Save2DSignal=2-D array (concatenate along first dimension)
  To Workspace6 : ToWorkspace  VariableName=Ts_t_dis  SampleTime=-1
      settings: Save2DSignal=2-D array (concatenate along first dimension)
  To Workspace7 : ToWorkspace  VariableName=Ah_dis  SampleTime=-1
      settings: Save2DSignal=2-D array (concatenate along first dimension)
  wires:
  2-D Lookup Table9/1 -> [C2_t_dis]
  [SoC_t] -> 2-D Lookup Table9/2
  Add18/1 -> [V_t], To Workspace2/1
  [V2_t] -> Scope35/1
  Cc1/1 -> Add17/2
  Divide1/1 -> Add20/1
  1-D Lookup Table1/1 -> [OCV_t]
  [SoC_t] -> Scope31/1
  Gain1/1 -> Integrator9/1
  [Tc_t] -> 2-D Lookup Table5/1
  [OCV_t] -> Add18/2
  Integrator10/1 -> To Workspace4/1, [V2_t]
  1/(Rc*Cc)1/1 -> Add17/1
  [R0_t_dis] -> Scope8/1
  Integrator4/1 -> To Workspace3/1, [V1_t]
  Divide4/1 -> Add2/1
  [Ts_t] -> Add19/1
  [C2_t_dis] -> Divide14/1, Divide1/2
  [V2_t] -> Divide14/3
  1/(Ru*Cs)1/1 -> Add14/1
  [SoC_t] -> 2-D Lookup Table8/2
  Add17/1 -> Integrator8/1
  [Tc_t] -> Scope36/1
  Constant1/1 -> Add16/1
  Divide12/1 -> [Q_t]
  2-D Lookup Table8/1 -> [C1_t_dis]
  Integrator7/1 -> To Workspace6/1, [Ts_t]
  1/(Rc*Cs)1/1 -> Add14/2
  [R1_t_dis] -> Scope11/1
  [Ts_t] -> Add16/2
  [V1_t] -> Add18/3
  Add16/1 -> 1/(Ru*Cs)1/1
  Add1/1 -> Divide12/1
  [I_t] -> Scope29/1
  Divide14/1 -> Add20/2
  [R2_t_dis] -> Divide14/2
  [Q_t] -> Scope30/1
  Add14/1 -> Integrator7/1
  Add2/1 -> Integrator4/1
  [Tc_t] -> 2-D Lookup Table7/1
  [V1_t] -> Scope34/1
  2-D Lookup Table7/1 -> [R2_t_dis]
  2-D Lookup Table6/1 -> [R1_t_dis]
  [V2_t] -> Add18/4
  [SoC_t] -> 2-D Lookup Table6/2
  [R2_t_dis] -> Scope18/1
  [SoC_t] -> 2-D Lookup Table5/2
  2-D Lookup Table5/1 -> [R0_t_dis]
  [OCV_t] -> To Workspace11/1, Scope32/1
  [Q_t] -> Cc1/1
  Divide3/1 -> Add2/2
  [I_t] -> Divide12/2
  Add19/1 -> 1/(Rc*Cc)1/1
  Add20/1 -> Integrator10/1
  [C1_t_dis] -> Scope19/1
  Divide2/1 -> Add18/1
  Add15/1 -> 1/(Rc*Cs)1/1
  [R1_t_dis] -> Divide3/2
  [C1_t_dis] -> Divide4/2, Divide3/1
  Integrator9/1 -> To Workspace/1, Scope2/1, [SoC_t]  "SoC_t"
  [Tc_t] -> Add15/2
  [OCV_t] -> Add1/2
  [C2_t_dis] -> Scope21/1
  [Tc_t] -> 2-D Lookup Table8/1
  [V1_t] -> Divide3/3
  [Tc_t] -> 2-D Lookup Table9/1
  [Ts_t] -> Add15/1
  [Ts_t] -> Scope37/1
  [V_t] -> Scope33/1
  [SoC_t] -> 1-D Lookup Table1/1
  [SoC_t] -> 2-D Lookup Table7/2
  [Tc_t] -> 2-D Lookup Table6/1
  [R0_t_dis] -> Divide2/1
  Integrator8/1 -> To Workspace5/1, [Tc_t]
  [V_t] -> Add1/1
  Constant10/1 -> Integrator4/2
  Constant4/1 -> Integrator7/2
  Constant9/1 -> Integrator10/2
  Constant3/1 -> Integrator8/2
  Integrator1/1 -> To Workspace7/1
  Gain2/1 -> Integrator1/1
  Constant5/1 -> MATLAB Function2/2(Cn)
  Constant6/1 -> MATLAB Function2/1(I_c)
  MATLAB Function2/1(I_t) -> To Workspace1/1, [I_t]
  [V_t] -> Compare To Constant1/1
  Compare To Constant1/1 -> Stop Simulation1/1
  [I_t] -> Gain1/1
  [Tc_t] -> Add19/2
  [I_t] -> Gain2/1
  [I_t] -> Divide4/1
  [I_t] -> Divide1/1
  [I_t] -> Divide2/2
  Constant7/1 -> Integrator9/2
  From34/1 -> 2-D Lookup Table1/1
  2-D Lookup Table1/1 -> Goto3/1
  Derivative/1 -> Divide/2
  Divide/1 -> Add18/5
  [I_t] -> Derivative/1
  L0/1 -> Divide/1
